simulink model "Finalmodel"  (R2018a)
settings: Solver=VariableStepAuto  StartTime=0.0  StopTime=100.0  RelTol=1e-3
settings Model: Creator=Arefin Mahin  LastModifiedBy=Arefin Mahin

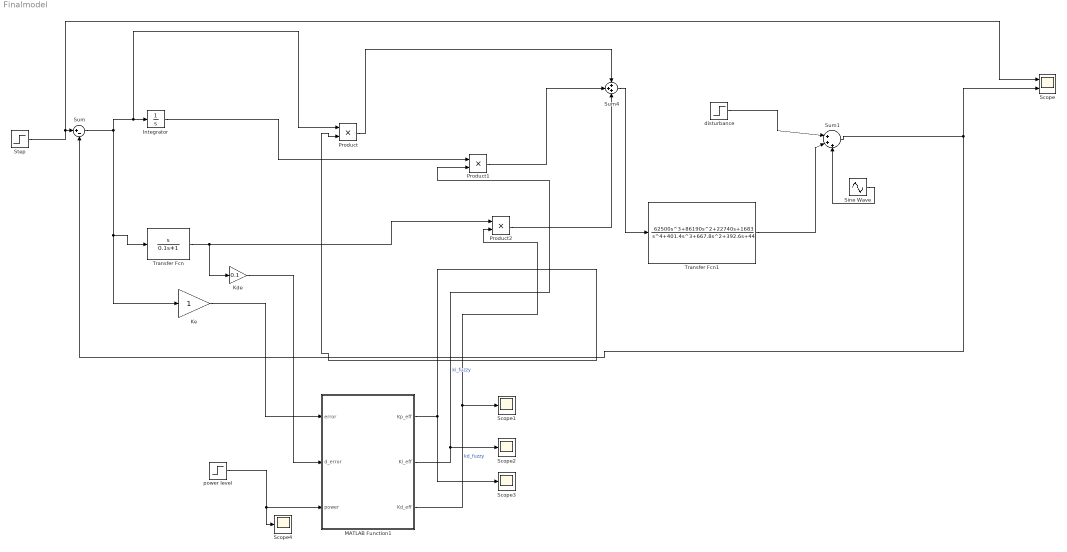
== system Finalmodel ==
  Integrator : Integrator
  Kde : Gain  Gain=0.1
  Ke : Gain
  MATLAB Function1 : MATLAB Function  TreatAsAtomicUnit=on
  Product : Product
  Product1 : Product
  Product2 : Product
  Scope : Scope  NumInputPorts=2
  Scope{1..4} (4 alike) : Scope
  Sine Wave : Sin  Frequency=2  SampleTime=0
  Step : Step  SampleTime=0
  Sum : Sum  Inputs=|+-
  Sum1 : Sum  Inputs=|+++
  Sum4 : Sum  Inputs=3
  Transfer Fcn : TransferFcn  Numerator=[1 0]  Denominator=[0.1 1]
  Transfer Fcn1 : TransferFcn  Numerator=[62500 86190 22740 1683]  Denominator=[1 401.4 667.8 392.6 44]
  disturbance : Step  Time=15  SampleTime=0
  power level : Step  Time=0  After=0.3  SampleTime=0
  wires:
  MATLAB Function1/1(Kp_eff) -> Scope3/1, Product/2
  Step/1 -> Scope/1, Sum/1
  Sum/1 -> Ke/1, Transfer Fcn/1, Product/1, Integrator/1
  Transfer Fcn1/1 -> Sum1/2
  Sum1/1 -> Scope/2, Sum/2
  disturbance/1 -> Sum1/1
  Integrator/1 -> Product1/1
  Product1/1 -> Sum4/2
  Product/1 -> Sum4/1
  Product2/1 -> Sum4/3
  Transfer Fcn/1 -> Product2/1, Kde/1
  Sum4/1 -> Transfer Fcn1/1
  MATLAB Function1/3(Kd_eff) -> Product2/2, Scope1/1  "kd_fuzzy"
  MATLAB Function1/2(Ki_eff) -> Product1/2, Scope2/1  "ki_fuzzy"
  Ke/1 -> MATLAB Function1/1(error)
  Kde/1 -> MATLAB Function1/2(d_error)
  power level/1 -> Scope4/1, MATLAB Function1/3(power)
  Sine Wave/1 -> Sum1/3

== matlab function Finalmodel/MATLAB Function1 ==
  settings: updateMethod=DISCRETE
  data: error input; Kp_eff output; d_error input; power input; Ki_eff output; Kd_eff output
function [Kp_eff, Ki_eff, Kd_eff] = fcn(error, d_error, power)
       %#codegen
       persistent W1 b1 W2 b2 W3 b3 sKp sKi sKd loaded
       if isempty(loaded)
           d  = coder.load('nn_weights_3in.mat');
           W1 = d.fc1_weight;  b1 = d.fc1_bias(:);
           W2 = d.fc2_weight;  b2 = d.fc2_bias(:);
           W3 = d.fc3_weight;  b3 = d.fc3_bias(:);
           s  = coder.load('scale_factors.mat');
           sKp = s.maxKp; sKi = s.maxKi; sKd = s.maxKd;
           loaded = true;
       end
       x  = [error; d_error; power];
       h1 = tanh(W1 * x  + b1);
       h2 = tanh(W2 * h1 + b2);
       y  = 1 ./ (1 + exp(-(W3 * h2 + b3)));
       Kp_eff = y(1) * sKp;
       Ki_eff = y(2) * sKi;
       Kd_eff = y(3) * sKd;
   end
